simulink model "Model"  (R2025b)
settings: Solver=ode45  StartTime=0.0  StopTime=10.0  MaxStep=1e-3  RelTol=1e-3
values from neighbouring files (symbols this model uses):
  alpha = m_p + m_c    (= 11)    [Coefficients.m]
  b = 2*zeta_c*omega_p*alpha    [Coefficients.m]
  beta = 2*zeta_p*omega_p*(lambda-mu^2/alpha)    [Coefficients.m]
  F_equilibrium = 1.5*alpha*g*tand(80)    [Coefficients.m]
  g = 9.80665    [Coefficients.m]
  lambda = 4/3 * m_p * l^2    (= 0.0133333333333)    [Coefficients.m]
  mu = m_p * l    (= 0.1)    [Coefficients.m]
  x_ref = 0    [Coefficients.m]
libraries: fuzblock x2
settings Model: SimulationMode=rapid-accelerator  Creator=barrios14101  LastModifiedBy=admin

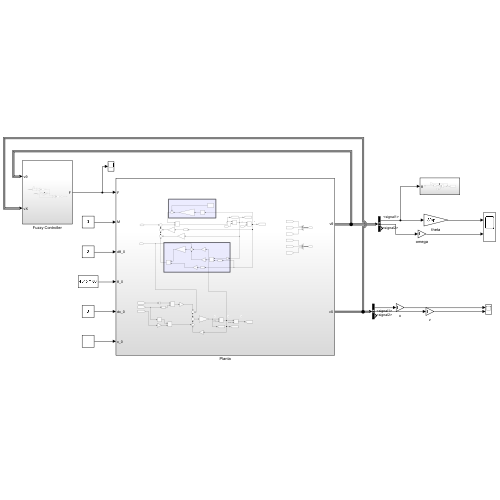
[thumbnail: Simulink's stored preview of the top-level diagram]
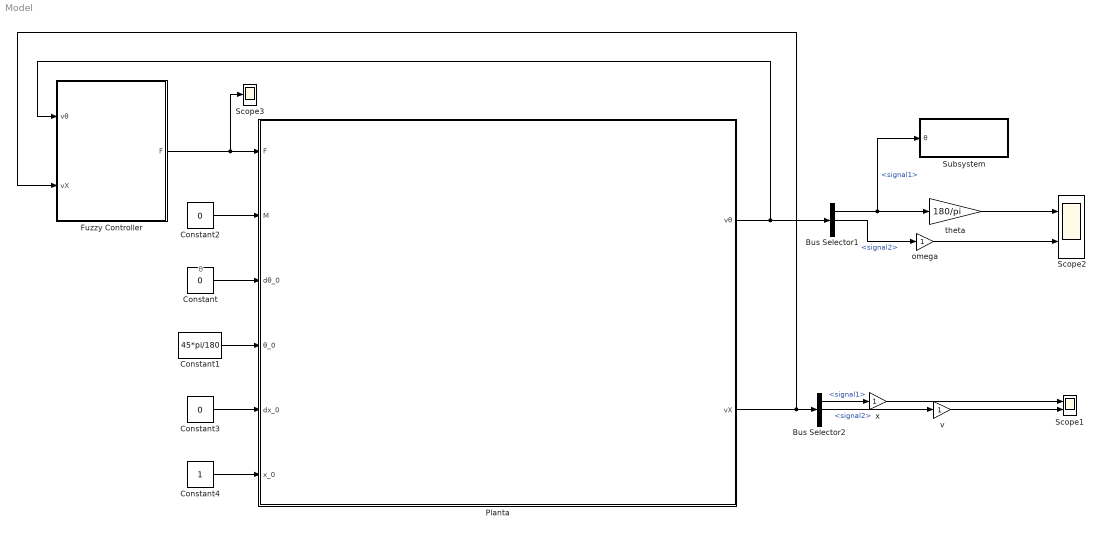
== system Model ==
  note: θ
  Bus Selector1 : BusSelector  OutputSignals=signal1,signal2,signal3
  Bus Selector2 : BusSelector  OutputSignals=signal1,signal2,signal3
  Constant : Constant  Value=0
  Constant1 : Constant  Value=45*pi/180
  Constant2 : Constant  Value=0
  Constant3 : Constant  Value=0
  Constant4 : Constant
  Fuzzy Controller : Subsystem
  Planta : Subsystem
  Scope1 : Scope  NumInputPorts=2
      settings: ActiveDisplayYMinimum=-2.2429215830298332  ActiveDisplayYMaximum=1.3603246203366481  DataLoggingDecimation=50
  Scope2 : Scope  NumInputPorts=2
      settings: ActiveDisplayYMinimum=-13.205630471505026  ActiveDisplayYMaximum=51.467292274611673  DataLoggingDecimation=50
  Scope3 : Scope
      settings: ActiveDisplayYMinimum=-600.8821467974509  ActiveDisplayYMaximum=220.63357171688955  DataLoggingDecimation=50  DataLoggingVariableName=ScopeData2
  Subsystem : Subsystem
  omega : Gain
  theta : Gain  Gain=180/pi
  v : Gain
  x : Gain
  wires:
  Planta/1(vθ) -> Fuzzy Controller/1(vθ), Bus Selector1/1
  Constant/1 -> Planta/3(dθ_0)
  Constant1/1 -> Planta/4(θ_0)
  Bus Selector1/1 -> Subsystem/1(θ), theta/1  "<signal1>"
  theta/1 -> Scope2/1
  Planta/2(vX) -> Fuzzy Controller/2(vX), Bus Selector2/1
  Bus Selector2/1 -> x/1  "<signal1>"
  Bus Selector1/2 -> omega/1  "<signal2>"
  Fuzzy Controller/1(F) -> Scope3/1, Planta/1(F)
  Constant2/1 -> Planta/2(M)
  Constant3/1 -> Planta/5(dx_0)
  Constant4/1 -> Planta/6(x_0)
  Bus Selector2/2 -> v/1  "<signal2>"
  omega/1 -> Scope2/2
  x/1 -> Scope1/1
  v/1 -> Scope1/2

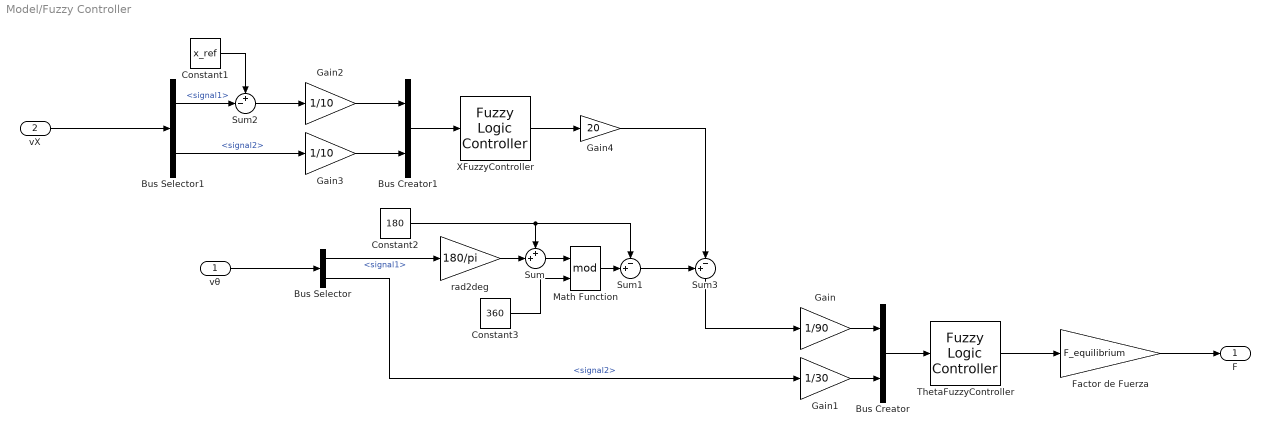
== system Model/Fuzzy Controller ==
  vθ : Inport
  vX : Inport  Port=2
  Bus Creator : BusCreator  Inputs=2
  Bus Creator1 : BusCreator  Inputs=2
  Bus Selector : BusSelector  OutputSignals=signal1,signal2
  Bus Selector1 : BusSelector  OutputSignals=signal1,signal2
  Constant1 : Constant  Value=x_ref
  Constant2 : Constant  Value=180
  Constant3 : Constant  Value=360
  Factor de Fuerza : Gain  Gain=F_equilibrium
  Gain : Gain  Gain=1/90
  Gain1 : Gain  Gain=1/30
  Gain2 : Gain  Gain=1/10
  Gain3 : Gain  Gain=1/10
  Gain4 : Gain  Gain=20
  Math Function : Math  Operator=mod  OutputSignalType=real
  Sum : Sum  Inputs=++|
  Sum1 : Sum  Inputs=-+|
  Sum2 : Sum  Inputs=+-|
  Sum3 : Sum  Inputs=+-|
  ThetaFuzzyController : fuzblock/Fuzzy Logic  Controller  FIS='ThetaFuzzyController.fis'  OutputSampleNumber=101  DataType=double  UseLookupTable=off  NumBreakpoints=10  FuzzifiedInputs=off  RuleFiringStrengths=off  RuleOutputs=off  AggregatedOutputs=off  SimulateUsing=Interpreted execution  OutOfRangeInputValueMessage=warning  NoRuleFiredMessage=warning  EmptyOutputFuzzySetMessage=warning
  XFuzzyController : fuzblock/Fuzzy Logic  Controller  FIS='XFuzzyController.fis'  OutputSampleNumber=101  DataType=double  UseLookupTable=off  NumBreakpoints=10  FuzzifiedInputs=off  RuleFiringStrengths=off  RuleOutputs=off  AggregatedOutputs=off  SimulateUsing=Interpreted execution  OutOfRangeInputValueMessage=warning  NoRuleFiredMessage=warning  EmptyOutputFuzzySetMessage=warning
  rad2deg : Gain  Gain=180/pi
  F : Outport
  wires:
  ThetaFuzzyController/1 -> Factor de Fuerza/1
  Constant2/1 -> Sum1/1, Sum/1
  rad2deg/1 -> Sum/2
  Math Function/1 -> Sum1/2
  Bus Selector/2 -> Gain1/1  "<signal2>"
  vθ/1 -> Bus Selector/1
  Bus Creator/1 -> ThetaFuzzyController/1
  Bus Selector/1 -> rad2deg/1  "<signal1>"
  Sum/1 -> Math Function/1
  Gain1/1 -> Bus Creator/2
  Constant3/1 -> Math Function/2
  Gain/1 -> Bus Creator/1
  vX/1 -> Bus Selector1/1
  Gain2/1 -> Bus Creator1/1
  Bus Selector1/2 -> Gain3/1  "<signal2>"
  Gain3/1 -> Bus Creator1/2
  Bus Creator1/1 -> XFuzzyController/1
  XFuzzyController/1 -> Gain4/1
  Sum1/1 -> Sum3/1
  Bus Selector1/1 -> Sum2/2  "<signal1>"
  Constant1/1 -> Sum2/1
  Sum2/1 -> Gain2/1
  Gain4/1 -> Sum3/2
  Sum3/1 -> Gain/1
  Factor de Fuerza/1 -> F/1

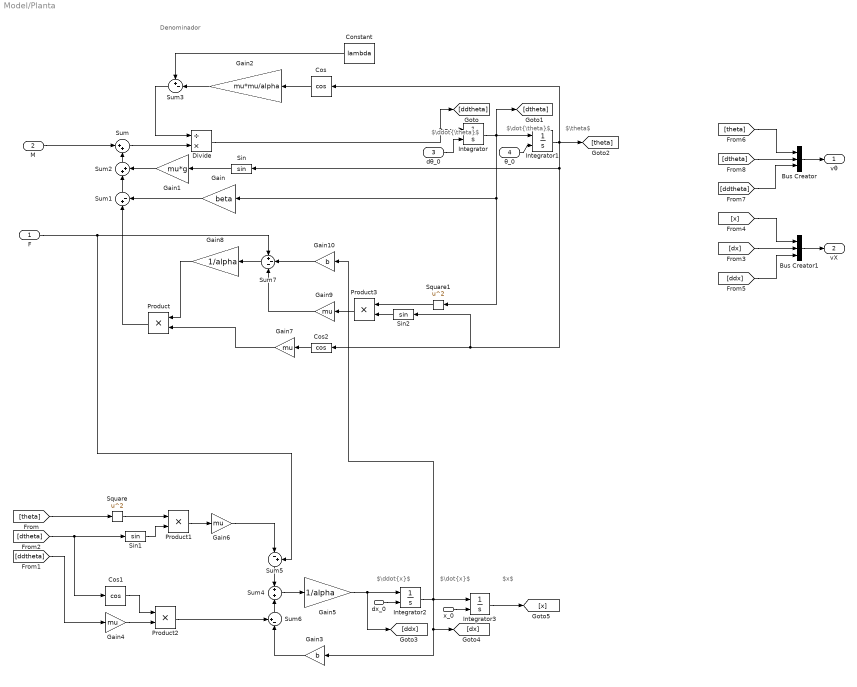
== system Model/Planta ==
  note: Denominador
  note: $\ddot{\theta}$
  note: $\dot{\theta}$
  note: $\theta$
  note: $x$
  note: $\ddot{x}$
  note: $\dot{x}$
  F : Inport
  M : Inport  Port=2
  dθ_0 : Inport  Port=3
  θ_0 : Inport  Port=4
  dx_0 : Inport  Port=5
  x_0 : Inport  Port=6
  Bus Creator : BusCreator  Inputs=3
  Bus Creator1 : BusCreator  Inputs=3
  Constant : Constant  Value=lambda
  Cos : Trigonometry  Operator=cos
  Cos1 : Trigonometry  Operator=cos
  Cos2 : Trigonometry  Operator=cos
  Divide : Product  Inputs=/*
  Gain : Gain  Gain=beta
  Gain1 : Gain  Gain=mu*g
  Gain10 : Gain  Gain=b
  Gain2 : Gain  Gain=mu*mu/alpha
  Gain3 : Gain  Gain=b
  Gain{4,6..7,9} (4 alike) : Gain  Gain=mu
  Gain5 : Gain  Gain=1/alpha
  Gain8 : Gain  Gain=1/alpha
  Integrator : Integrator  InitialConditionSource=external
  Integrator1 : Integrator  InitialConditionSource=external  InitialCondition=pi/12
  Integrator2 : Integrator  InitialConditionSource=external
  Integrator3 : Integrator  InitialConditionSource=external
  Product{,1..3} (4 alike) : Product
  Sin : Trigonometry
  Sin1 : Trigonometry
  Sin2 : Trigonometry
  Square : Math  Operator=square
  Square1 : Math  Operator=square
  Sum : Sum  Inputs=|++
  Sum1 : Sum  Inputs=|+-
  Sum2 : Sum  Inputs=|++
  Sum3 : Sum  Inputs=+-|
  Sum4 : Sum
  Sum5 : Sum  Inputs=|-+
  Sum6 : Sum  Inputs=+-|
  Sum7 : Sum  Inputs=+--
  vθ : Outport
  vX : Outport  Port=2
  wires:
  Gain8/1 -> Product/1
  Product2/1 -> Sum6/1
  Sum5/1 -> Sum4/1
  Sum6/1 -> Sum4/2
  Constant/1 -> Sum3/1
  Sum1/1 -> Sum2/1
  M/1 -> Sum/1
  Gain3/1 -> Sum6/2
  Gain7/1 -> Product/2
  Sum2/1 -> Sum/2
  F/1 -> Sum5/2, Sum7/1
  Integrator2/1 -> Gain10/1, Integrator3/1, Gain3/1, [dx]
  Gain/1 -> Sum1/2
  [theta] -> Square/1
  Sum7/1 -> Gain8/1
  Square1/1 -> Product3/1
  Gain6/1 -> Sum5/1
  Integrator1/1 -> Sin/1, Sin2/1, Cos2/1, [theta], Cos/1
  Gain4/1 -> Product2/2
  Divide/1 -> [ddtheta], Integrator/1
  Cos/1 -> Gain2/1
  [ddtheta] -> Gain4/1
  Sum/1 -> Divide/2
  Integrator/1 -> [dtheta], Square1/1, Gain/1, Integrator1/1
  Gain1/1 -> Sum2/2
  Gain5/1 -> [ddx], Integrator2/1
  Gain2/1 -> Sum3/2
  Gain9/1 -> Sum7/3
  Cos2/1 -> Gain7/1
  Cos1/1 -> Product2/1
  Sum4/1 -> Gain5/1
  Integrator3/1 -> [x]
  Sin1/1 -> Product1/2
  [dtheta] -> Cos1/1, Sin1/1
  Product3/1 -> Gain9/1
  Gain10/1 -> Sum7/2
  Sum3/1 -> Divide/1
  Product1/1 -> Gain6/1
  Product/1 -> Sum1/1
  Sin2/1 -> Product3/2
  Square/1 -> Product1/1
  Sin/1 -> Gain1/1
  [dtheta] -> Bus Creator/2
  [ddtheta] -> Bus Creator/3
  [x] -> Bus Creator1/1
  [dx] -> Bus Creator1/2
  [ddx] -> Bus Creator1/3
  Bus Creator/1 -> vθ/1
  Bus Creator1/1 -> vX/1
  [theta] -> Bus Creator/1
  dθ_0/1 -> Integrator/2
  θ_0/1 -> Integrator1/2
  dx_0/1 -> Integrator2/2
  x_0/1 -> Integrator3/2

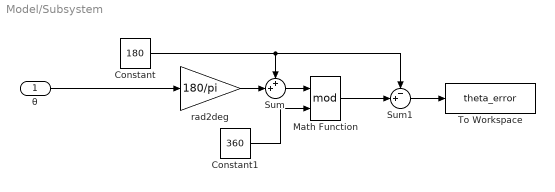
== system Model/Subsystem ==
  θ : Inport
  Constant : Constant  Value=180
  Constant1 : Constant  Value=360
  Math Function : Math  Operator=mod  OutputSignalType=real
  Sum : Sum  Inputs=++|
  Sum1 : Sum  Inputs=-+|
  To Workspace : ToWorkspace  VariableName=theta_error  SaveFormat=Timeseries  SampleTime=-1
  rad2deg : Gain  Gain=180/pi
  wires:
  Math Function/1 -> Sum1/2
  rad2deg/1 -> Sum/2
  Sum/1 -> Math Function/1
  Constant/1 -> Sum1/1, Sum/1
  θ/1 -> rad2deg/1
  Constant1/1 -> Math Function/2
  Sum1/1 -> To Workspace/1
